simulink model "feedforward"  (R2017b)
settings: Solver=VariableStepAuto  StartTime=0.0  StopTime=37  RelTol=1e-3
libraries: roblocks x3
settings Model: Creator=ArsalanBangash  LastModifiedBy=ArsalanBangash

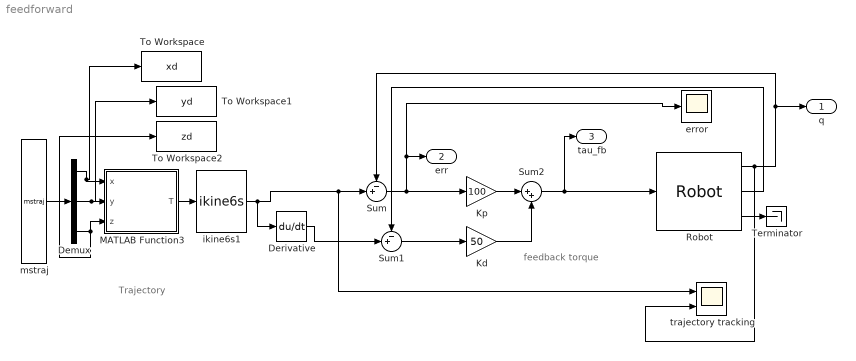
== system feedforward ==
  note: feedback torque
  note: Trajectory
  Demux : Demux  Outputs=3
  Derivative : Derivative
  Kd : Gain  Gain=50  SaturateOnIntegerOverflow=on  OutDataTypeStr=Inherit: Same as input  ParamDataTypeStr=Inherit: Same as input
  Kp : Gain  Gain=100  SaturateOnIntegerOverflow=on  OutDataTypeStr=Inherit: Same as input  ParamDataTypeStr=Inherit: Same as input
  MATLAB Function3 : MATLAB Function  TreatAsAtomicUnit=on
  Robot : roblocks/Arm/Robot  robot=p560.nofriction  q0=[0 0 0 0 0 0]
  Sum : Sum  Inputs=-+|  SaturateOnIntegerOverflow=on  InputSameDT=on  OutDataTypeStr=Inherit: Same as first input
  Sum1 : Sum  Inputs=-+|  SaturateOnIntegerOverflow=on  InputSameDT=on  OutDataTypeStr=Inherit: Same as first input
  Sum2 : Sum  Inputs=|++  SaturateOnIntegerOverflow=on  InputSameDT=on  OutDataTypeStr=Inherit: Same as first input
  Terminator : Terminator
  To Workspace : ToWorkspace  VariableName=xd  SampleTime=-1
  To Workspace1 : ToWorkspace  VariableName=yd  SampleTime=-1
  To Workspace2 : ToWorkspace  VariableName=zd  SampleTime=-1
  error : Scope
  ikine6s1 : roblocks/Arm/ikine6s  robot=p560  conf='luf'
  mstraj : roblocks/Toolbox/mstraj  path=|  vaxis=[0.1 0.1 0.1]  tseg=[]  dt=0.1  tacc=0  setsimtime=on
      | [ 0.5,-0.5,0.1;
      |  0.5,-0.5,0.5 ;0.5,0.5,0.5;0.5,0.5,0.1; 0.5,-0.5,0.1; 0.5,-0.5,0.5; 0.5 0 0]
  "trajectory tracking " : Scope  NumInputPorts=2
  q : Outport
  err : Outport  Port=2
  tau_fb : Outport  Port=3
  wires:
  Kd/1 -> Sum2/2
  Robot/1 -> "trajectory tracking "/2, q/1, Sum/1
  Robot/2 -> Sum1/1
  Robot/3 -> Terminator/1
  Derivative/1 -> Sum1/2
  Kp/1 -> Sum2/1
  Sum2/1 -> Robot/1, tau_fb/1
  Sum1/1 -> Kd/1
  ikine6s1/1 -> Derivative/1, "trajectory tracking "/1, Sum/2
  Sum/1 -> error/1, err/1, Kp/1
  MATLAB Function3/1(T) -> ikine6s1/1
  Demux/2 -> To Workspace1/1, MATLAB Function3/2(y)
  Demux/1 -> To Workspace/1, MATLAB Function3/1(x)
  mstraj/1 -> Demux/1
  Demux/3 -> MATLAB Function3/3(z), To Workspace2/1

== matlab function feedforward/MATLAB Function3 ==
  data: x input; T output; y input; z input
function T = fcn(x,y,z)

T=transl(x,y,z);
